simulink model "model6"  (R2022a)
settings: Solver=FixedStepAuto  StartTime=0.0  StopTime=2  FixedStep=1e-5  RelTol=1e-3
model workspace (MAT data in the model file):
  b1 = 10
  b2 = 1500
  downSpringHeight = 10
  g = 9.81
  groundHeight = 100
  k1 = 400
  k2 = 10000000
  m1 = 3.6
  m1IniHeight = 10
  m2 = 3.6
  m3 = 3.6
  upSpringHeight = 10
settings Model: Creator=Tsing  LastModifiedBy=whatastarrynight

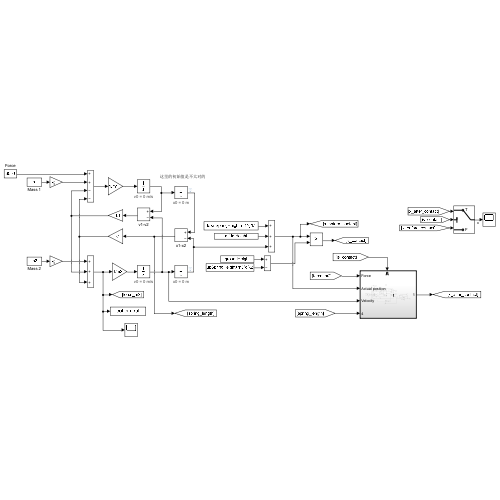
[thumbnail: Simulink's stored preview of the top-level diagram]
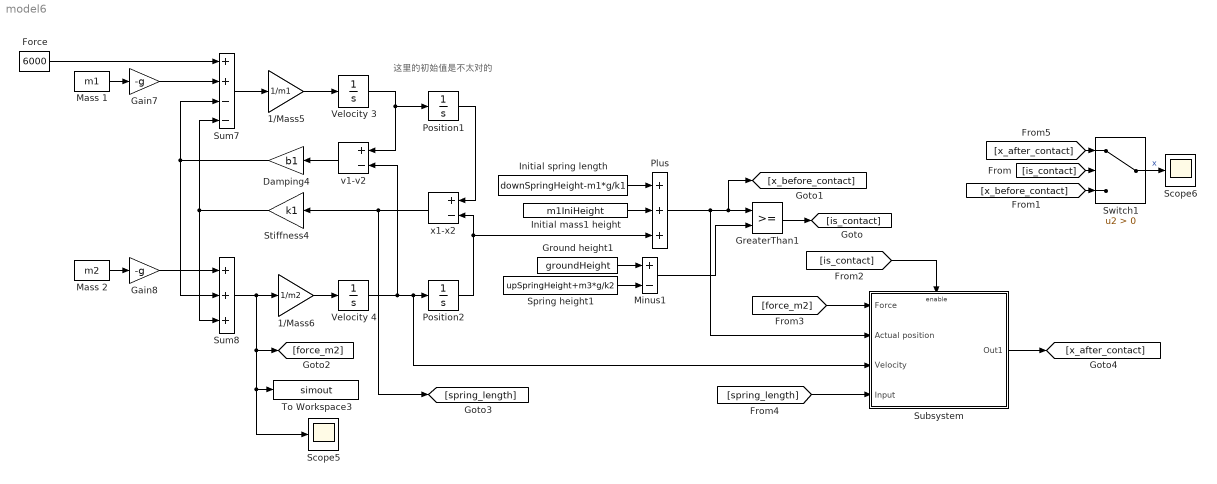
== system model6 ==
  note: 这里的初始值是不太对的
  1/Mass5 : Gain  Gain=1/m1  SaturateOnIntegerOverflow=on  OutDataTypeStr=Inherit: Same as input  ParamDataTypeStr=Inherit: Same as input
  1/Mass6 : Gain  Gain=1/m2  SaturateOnIntegerOverflow=on  OutDataTypeStr=Inherit: Same as input  ParamDataTypeStr=Inherit: Same as input
  Damping4 : Gain  Gain=b1  SaturateOnIntegerOverflow=on  OutDataTypeStr=Inherit: Same as input  ParamDataTypeStr=Inherit: Same as input
  Force : Constant  Value=6000
  Gain7 : Gain  Gain=-g
  Gain8 : Gain  Gain=-g
  GreaterThan1 : RelationalOperator  OutDataTypeStr=boolean  RndMeth=Simplest  InputSameDT=off
  Ground height1 : Constant  Value=groundHeight
  Initial mass1 height : Constant  Value=m1IniHeight
  Initial spring length : Constant  Value=downSpringHeight-m1*g/k1
  Mass 1 : Constant  Value=m1
  Mass 2 : Constant  Value=m2
  Minus1 : Sum  Inputs=+-
  Plus : Sum  Inputs=+++
  Position1 : Integrator
      settings: AttributesFormatString=x0 = %<InitialCondition> m
  Position2 : Integrator
      settings: AttributesFormatString=x0 = %<InitialCondition> m
  Scope5 : Scope
  Scope6 : Scope
  Spring height1 : Constant  Value=upSpringHeight+m3*g/k2
  Stiffness4 : Gain  Gain=k1  SaturateOnIntegerOverflow=on  OutDataTypeStr=Inherit: Same as input  ParamDataTypeStr=Inherit: Same as input
  Subsystem : Subsystem
  Sum7 : Sum  Inputs=++--  InputSameDT=on  SaturateOnIntegerOverflow=on  OutDataTypeStr=Inherit: Same as first input
  Sum8 : Sum  Inputs=+++  InputSameDT=on  SaturateOnIntegerOverflow=on  OutDataTypeStr=Inherit: Same as first input
  Switch1 : Switch  Criteria=u2 > Threshold  SaturateOnIntegerOverflow=off  InputSameDT=off
  To Workspace3 : ToWorkspace  VariableName=simout  SaveFormat=Timeseries  SampleTime=-1
  Velocity 3 : Integrator
      settings: AttributesFormatString=v0 = %<InitialCondition> m/s
  Velocity 4 : Integrator
      settings: AttributesFormatString=v0 = %<InitialCondition> m/s
  v1-v2 : Sum  Inputs=+-
  x1-x2 : Sum  Inputs=+-
  wires:
  Gain8/1 -> Sum8/1
  Mass 2/1 -> Gain8/1
  Sum8/1 -> [force_m2], Scope5/1, To Workspace3/1, 1/Mass6/1
  Stiffness4/1 -> Sum7/4, Sum8/3
  Velocity 3/1 -> Position1/1, v1-v2/1
  Damping4/1 -> Sum7/3, Sum8/2
  Force/1 -> Sum7/1
  v1-v2/1 -> Damping4/1
  1/Mass5/1 -> Velocity 3/1
  Sum7/1 -> 1/Mass5/1
  Velocity 4/1 -> Subsystem/3(Velocity), Position2/1, v1-v2/2
  Position1/1 -> x1-x2/1
  1/Mass6/1 -> Velocity 4/1
  Mass 1/1 -> Gain7/1
  Gain7/1 -> Sum7/2
  Position2/1 -> Plus/3, x1-x2/2
  Spring height1/1 -> Minus1/2
  Ground height1/1 -> Minus1/1
  Initial spring length/1 -> Plus/1
  Minus1/1 -> GreaterThan1/2
  Initial mass1 height/1 -> Plus/2
  [is_contact] -> Switch1/2
  Switch1/1 -> Scope6/1  "x"
  [is_contact] -> Subsystem/Enable
  [force_m2] -> Subsystem/1(Force)
  [spring_length] -> Subsystem/4(Input)
  Subsystem/1(Out1) -> [x_after_contact]
  [x_after_contact] -> Switch1/1
  x1-x2/1 -> [spring_length], Stiffness4/1
  GreaterThan1/1 -> [is_contact]
  [x_before_contact] -> Switch1/3
  Plus/1 -> Subsystem/2(Actual position), [x_before_contact], GreaterThan1/1

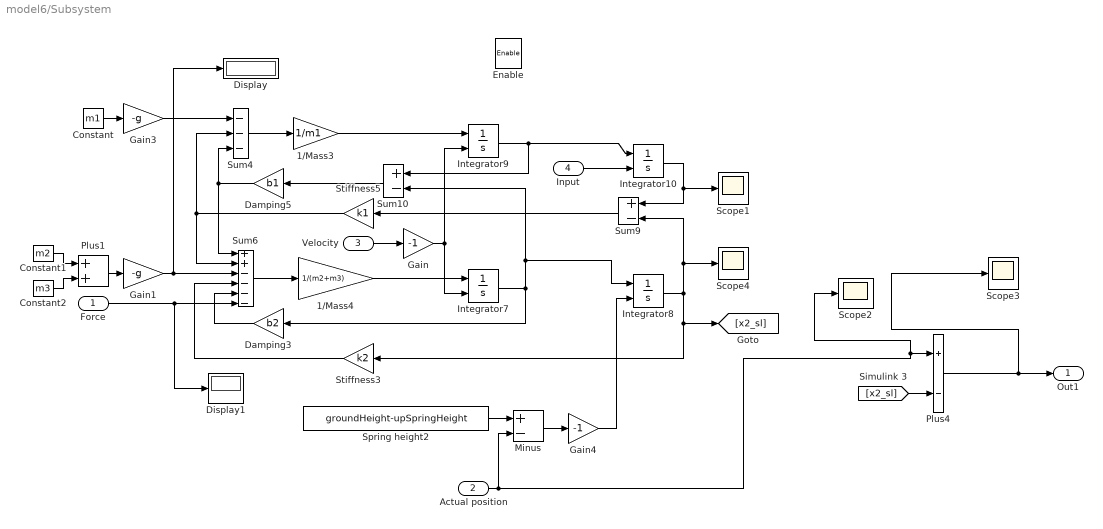
== system model6/Subsystem ==
  Force : Inport
  Actual position : Inport  Port=2
  Velocity : Inport  Port=3
  Input : Inport  Port=4
  Enable : EnablePort
  1/Mass3 : Gain  Gain=1/m1  SaturateOnIntegerOverflow=on  OutDataTypeStr=Inherit: Same as input  ParamDataTypeStr=Inherit: Same as input
  1/Mass4 : Gain  Gain=1/(m2+m3)  SaturateOnIntegerOverflow=on  OutDataTypeStr=Inherit: Same as input  ParamDataTypeStr=Inherit: Same as input
  Constant : Constant  Value=m1
  Constant1 : Constant  Value=m2
  Constant2 : Constant  Value=m3
  Damping3 : Gain  Gain=b2  SaturateOnIntegerOverflow=on  OutDataTypeStr=Inherit: Same as input  ParamDataTypeStr=Inherit: Same as input
  Damping5 : Gain  Gain=b1  SaturateOnIntegerOverflow=on  OutDataTypeStr=Inherit: Same as input  ParamDataTypeStr=Inherit: Same as input
  Display : Display
  Display1 : Display
  Gain : Gain  Gain=-1
  Gain1 : Gain  Gain=-g
  Gain3 : Gain  Gain=-g
  Gain4 : Gain  Gain=-1
  Integrator{7..10} (4 alike) : Integrator  InitialConditionSource=external
      Integrator10 settings: AttributesFormatString=x0 = %<InitialCondition> m
      Integrator7 settings: AttributesFormatString=v0 = %<InitialCondition> m/s
      Integrator8 settings: AttributesFormatString=x0 = %<InitialCondition> m
      Integrator9 settings: AttributesFormatString=v0 = %<InitialCondition> m/s
  Minus : Sum  Inputs=+-
  Plus1 : Sum
  Plus4 : Sum  Inputs=+-
  Scope{1..4} (4 alike) : Scope
  Spring height2 : Constant  Value=groundHeight-upSpringHeight
  Stiffness3 : Gain  Gain=k2  SaturateOnIntegerOverflow=on  OutDataTypeStr=Inherit: Same as input  ParamDataTypeStr=Inherit: Same as input
  Stiffness5 : Gain  Gain=k1  SaturateOnIntegerOverflow=on  OutDataTypeStr=Inherit: Same as input  ParamDataTypeStr=Inherit: Same as input
  Sum10 : Sum  Inputs=+-  InputSameDT=on  SaturateOnIntegerOverflow=on  OutDataTypeStr=Inherit: Same as first input
  Sum4 : Sum  Inputs=---  InputSameDT=on  SaturateOnIntegerOverflow=on  OutDataTypeStr=Inherit: Same as first input
  Sum6 : Sum  Inputs=++----  InputSameDT=on  SaturateOnIntegerOverflow=on  OutDataTypeStr=Inherit: Same as first input
  Sum9 : Sum  Inputs=+-  InputSameDT=on  SaturateOnIntegerOverflow=on  OutDataTypeStr=Inherit: Same as first input
  Out1 : Outport
  wires:
  Integrator9/1 -> Integrator10/1, Sum10/1
  Integrator10/1 -> Sum9/1, Scope1/1
  Force/1 -> Display1/1, Sum6/6
  1/Mass4/1 -> Integrator7/1
  Integrator7/1 -> Damping3/1, Sum10/2, Integrator8/1
  Damping5/1 -> Sum4/3, Sum6/1
  Damping3/1 -> Sum6/5
  Constant2/1 -> Plus1/2
  Stiffness3/1 -> Sum6/4
  Sum10/1 -> Damping5/1
  1/Mass3/1 -> Integrator9/1
  Constant/1 -> Gain3/1
  Constant1/1 -> Plus1/1
  Sum4/1 -> 1/Mass3/1
  Sum6/1 -> 1/Mass4/1
  Stiffness5/1 -> Sum6/2, Sum4/2
  Gain1/1 -> Display/1, Sum6/3
  Sum9/1 -> Stiffness5/1
  Plus1/1 -> Gain1/1
  Actual position/1 -> Minus/2, Scope2/1, Plus4/1
  [x2_sl] -> Plus4/2
  Velocity/1 -> Gain/1
  Gain/1 -> Integrator9/2, Integrator7/2
  Plus4/1 -> Scope3/1, Out1/1
  Gain4/1 -> Integrator8/2
  Gain3/1 -> Sum4/1
  Input/1 -> Integrator10/2
  Integrator8/1 -> Scope4/1, Sum9/2, Stiffness3/1, [x2_sl]
  Spring height2/1 -> Minus/1
  Minus/1 -> Gain4/1
